simulink model "hnn_2_neurons"  (R2024b)
settings: Solver=VariableStepAuto  StartTime=0.0  StopTime=10  RelTol=1e-3
settings Model: Creator=merlin  LastModifiedBy=merlin

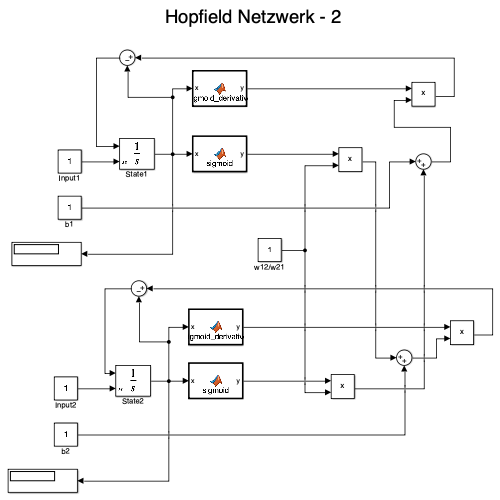
[thumbnail: Simulink's stored preview of the top-level diagram]
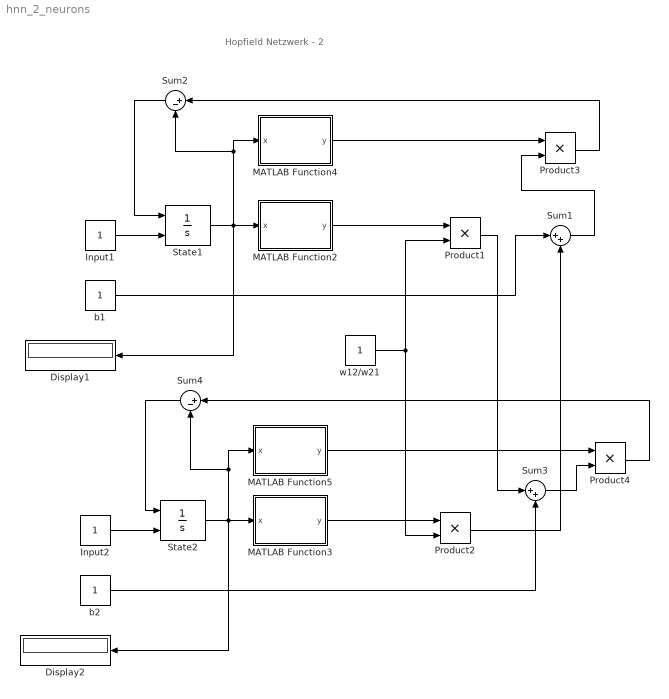
== system hnn_2_neurons ==
  note: Hopfield Netzwerk - 2
  Display1 : Display
  Display2 : Display
  Input1 : Constant
  Input2 : Constant
  MATLAB Function2 : MATLAB Function  TreatAsAtomicUnit=on
  MATLAB Function3 : MATLAB Function  TreatAsAtomicUnit=on
  MATLAB Function4 : MATLAB Function  TreatAsAtomicUnit=on
  MATLAB Function5 : MATLAB Function  TreatAsAtomicUnit=on
  Product{1..4} (4 alike) : Product
  State1 : Integrator  InitialConditionSource=external
  State2 : Integrator  InitialConditionSource=external
  Sum1 : Sum  Inputs=|++
  Sum2 : Sum  Inputs=|+-
  Sum3 : Sum  Inputs=|++
  Sum4 : Sum  Inputs=|+-
  b1 : Constant
  b2 : Constant
  w12/w21 : Constant
  wires:
  Input1/1 -> State1/2
  State1/1 -> Display1/1, Sum2/2, MATLAB Function4/1(x), MATLAB Function2/1(x)
  Input2/1 -> State2/2
  State2/1 -> Display2/1, Sum4/2, MATLAB Function5/1(x), MATLAB Function3/1(x)
  MATLAB Function2/1(y) -> Product1/1
  MATLAB Function3/1(y) -> Product2/1
  w12/w21/1 -> Product2/2, Product1/2
  Product2/1 -> Sum1/2
  b1/1 -> Sum1/1
  Sum1/1 -> Product3/2
  MATLAB Function4/1(y) -> Product3/1
  Product3/1 -> Sum2/1
  Sum2/1 -> State1/1
  Product1/1 -> Sum3/1
  b2/1 -> Sum3/2
  MATLAB Function5/1(y) -> Product4/1
  Sum3/1 -> Product4/2
  Product4/1 -> Sum4/1
  Sum4/1 -> State2/1

== matlab function hnn_2_neurons/MATLAB Function3 ==
  data: x input; y output
function y = sigmoid(x)
y = 1 ./ (1 + exp(-x));
end

== matlab function hnn_2_neurons/MATLAB Function4 ==
  data: x input; y output
function y = sigmoid_derivative(x)
sigmoid = 1 ./ (1 + exp(-x));
y = sigmoid .* (1 - sigmoid);
end

== matlab function hnn_2_neurons/MATLAB Function5 ==
  data: x input; y output
function y = sigmoid_derivative(x)
sigmoid = 1 ./ (1 + exp(-x));
y = sigmoid .* (1 - sigmoid);
end

== matlab function hnn_2_neurons/MATLAB Function2 ==
  data: x input; y output
function y = sigmoid(x)
y = 1 ./ (1 + exp(-x));
end
